simulink model "QCwithActDyn_seperate_channels"  (R2019b)
settings: Solver=FixedStepAuto  StartTime=0.0  StopTime=10  FixedStep=0.001  RelTol=1e-3
model workspace (MAT data in the model file):
  time_step = 0.01
libraries: simulink x1
settings Model: Creator=Abdulaziz Y. Alkayas  LastModifiedBy=aaa_b
settings SolverCC: SolverResetMethod=Robust
settings DebuggingCC: ArithmeticOperatorsInVariantConditions=warning
settings HardwareCC: TargetBitPerPointer=64  TargetBitPerSizeT=64  TargetBitPerPtrDiffT=64  TargetLongLongMode=on  TargetIntDivRoundTo=Zero  TargetEndianess=LittleEndian  TargetWordSize=64  TargetHWDeviceType=MATLAB Host  ProdEqTarget=off
settings SFSimCC: CustomCodeUndefinedFunction=UseInterfaceOnly
settings RTWCC: Description=Generic Real-Time Target

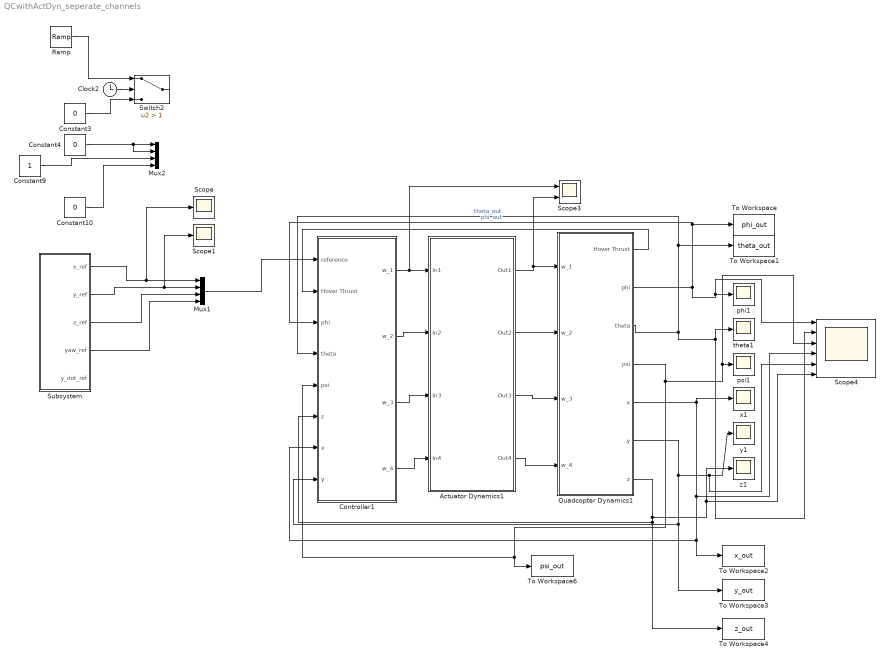
== system QCwithActDyn_seperate_channels ==
  Actuator Dynamics1 : Subsystem
  Clock2 : Clock
  Constant10 : Constant  Value=0
  Constant3 : Constant  Value=0
  Constant4 : Constant  Value=0
  Constant9 : Constant
  Controller1 : Subsystem
  Mux1 : Mux
  Mux2 : Mux
  Quadcopter Dynamics1 : Subsystem
  Ramp : simulink/Sources/Ramp  slope=1  start=2  InitialOutput=0
  Scope : Scope
  Scope1 : Scope
  Scope3 : Scope  NumInputPorts=2
  Scope4 : Scope  NumInputPorts=6
  Subsystem : Subsystem
  Switch2 : Switch  Criteria=u2 > Threshold  Threshold=1
  To Workspace : ToWorkspace  VariableName=phi_out  SaveFormat=Timeseries  SampleTime=-1
  To Workspace1 : ToWorkspace  VariableName=theta_out  SaveFormat=Timeseries  SampleTime=-1
  To Workspace2 : ToWorkspace  VariableName=x_out  SaveFormat=Timeseries  SampleTime=-1
  To Workspace3 : ToWorkspace  VariableName=y_out  SaveFormat=Timeseries  SampleTime=-1
  To Workspace4 : ToWorkspace  VariableName=z_out  SaveFormat=Timeseries  SampleTime=-1
  To Workspace6 : ToWorkspace  VariableName=psi_out  SaveFormat=Timeseries  SampleTime=-1
  phi1 : Scope
  psi1 : Scope
  theta1 : Scope
  x1 : Scope
  y1 : Scope
  z1 : Scope
  wires:
  Actuator Dynamics1/4(Out4) -> Quadcopter Dynamics1/4(w_4)
  Actuator Dynamics1/3(Out3) -> Quadcopter Dynamics1/3(w_3)
  Actuator Dynamics1/2(Out2) -> Quadcopter Dynamics1/2(w_2)
  Actuator Dynamics1/1(Out1) -> Scope3/2, Quadcopter Dynamics1/1(w_1)
  Controller1/4(w_4) -> Actuator Dynamics1/4(In4)
  Controller1/3(w_3) -> Actuator Dynamics1/3(In3)
  Controller1/2(w_2) -> Actuator Dynamics1/2(In2)
  Controller1/1(w_1) -> Actuator Dynamics1/1(In1), Scope3/1
  Quadcopter Dynamics1/3(theta) -> theta1/1, Scope4/2, To Workspace1/1, Controller1/4(theta)  "theta_out"
  Quadcopter Dynamics1/2(phi) -> Controller1/3(phi), To Workspace/1, phi1/1, Scope4/1  "phi_out"
  Quadcopter Dynamics1/4(psi) -> To Workspace6/1, Controller1/5(psi), psi1/1, Scope4/3
  Quadcopter Dynamics1/7(z) -> To Workspace4/1, Controller1/6(z), z1/1, Scope4/6
  Quadcopter Dynamics1/1(Hover Thrust) -> Controller1/2(Hover Thrust)
  Quadcopter Dynamics1/5(x) -> x1/1, Scope4/4, To Workspace2/1, Controller1/7(x)
  Quadcopter Dynamics1/6(y) -> To Workspace3/1, Controller1/8(y), y1/1, Scope4/5
  Ramp/1 -> Switch2/1
  Constant9/1 -> Mux2/3
  Constant10/1 -> Mux2/4
  Clock2/1 -> Switch2/2
  Constant3/1 -> Switch2/3
  Subsystem/3("z_ref ") -> Mux1/3
  Subsystem/4("yaw_ref ") -> Mux1/4
  Subsystem/1("x_ref ") -> Mux1/1, Scope/1
  Subsystem/2("y_ref ") -> Mux1/2, Scope1/1
  Constant4/1 -> Mux2/2, Mux2/1
  Mux1/1 -> Controller1/1(reference)

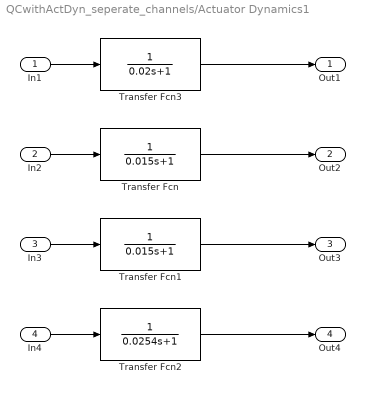
== system QCwithActDyn_seperate_channels/Actuator Dynamics1 ==
  In1 : Inport
  In2 : Inport  Port=2
  In3 : Inport  Port=3
  In4 : Inport  Port=4
  Transfer Fcn : TransferFcn  Denominator=[0.015 1]
  Transfer Fcn1 : TransferFcn  Denominator=[0.015 1]
  Transfer Fcn2 : TransferFcn  Denominator=[0.0254 1]
  Transfer Fcn3 : TransferFcn  Denominator=[0.02 1]
  Out1 : Outport
  Out2 : Outport  Port=2
  Out3 : Outport  Port=3
  Out4 : Outport  Port=4
  wires:
  In1/1 -> Transfer Fcn3/1
  In3/1 -> Transfer Fcn1/1
  Transfer Fcn3/1 -> Out1/1
  Transfer Fcn/1 -> Out2/1
  In2/1 -> Transfer Fcn/1
  Transfer Fcn1/1 -> Out3/1
  Transfer Fcn2/1 -> Out4/1
  In4/1 -> Transfer Fcn2/1

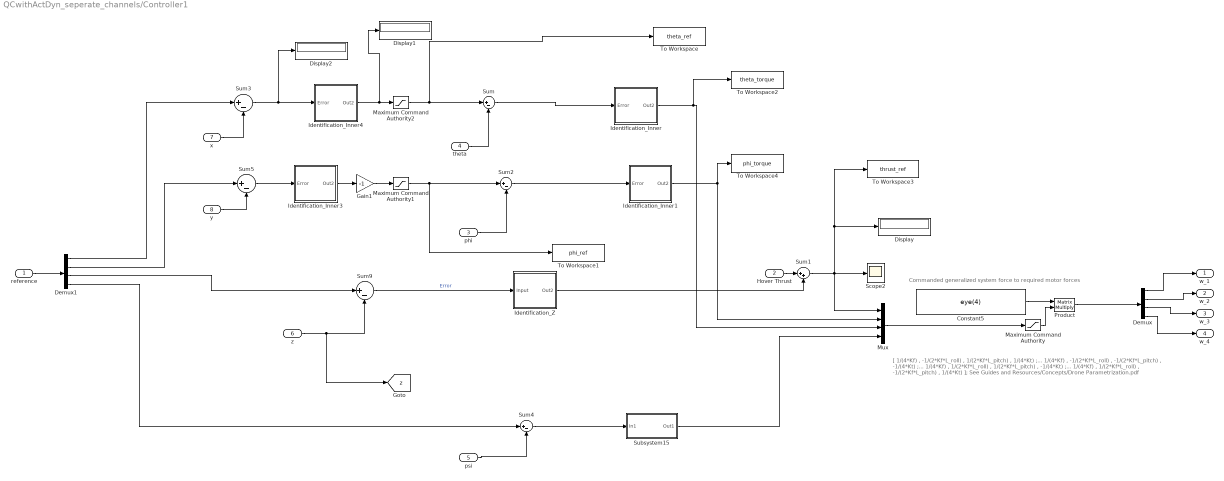
== system QCwithActDyn_seperate_channels/Controller1 ==
  note: [ 1/(4*Kf) , -1/(2*Kf*L_roll) , 1/(2*Kf*L_pitch) , 1/(4*Kt) ;...
      | 1/(4*Kf) , -1/(2*Kf*L_roll) , -1/(2*Kf*L_pitch) , -1/(4*Kt) ;...
      | 1/(4*Kf) , 1/(2*Kf*L_roll) , 1/(2*Kf*L_pitch) , -1/(4*Kt) ;...
      | 1/(4*Kf) , 1/(2*Kf*L_roll) , -1/(2*Kf*L_pitch) , 1/(4*Kt) ];
      |
      | See Guides and Resources/Concepts/Drone Parametrization.pdf
  note: Commanded generalized system force to required motor forces
  reference : Inport
  Hover Thrust : Inport  Port=2
  phi : Inport  Port=3
  theta : Inport  Port=4
  psi : Inport  Port=5
  z : Inport  Port=6
  x : Inport  Port=7
  y : Inport  Port=8
  Constant5 : Constant  Value=eye(4)
  Demux : Demux
  Demux1 : Demux
  Display : Display
  Display1 : Display
  Display2 : Display
  Gain1 : Gain  Gain=-1
  Identification_Inner : Subsystem
  Identification_Inner1 : Subsystem
  Identification_Inner3 : Subsystem
  Identification_Inner4 : Subsystem
  Identification_Z : Subsystem
  Maximum Command Authority : Saturate  UpperLimit=[Inf Inf Inf Inf]  LowerLimit=[-inf -Inf -Inf -Inf]
  Maximum Command Authority1 : Saturate  UpperLimit=pi/2  LowerLimit=-pi/2
  Maximum Command Authority2 : Saturate  UpperLimit=pi/2  LowerLimit=-pi/2
  Mux : Mux
  Product : Product  Multiplication=Matrix(*)
  Scope2 : Scope
  Subsystem15 : Subsystem
  Sum{,2..5,9} (6 alike) : Sum  Inputs=|+-
  Sum1 : Sum  Inputs=|++
  To Workspace : ToWorkspace  VariableName=theta_ref  SaveFormat=Timeseries  SampleTime=-1
  To Workspace1 : ToWorkspace  VariableName=phi_ref  SaveFormat=Timeseries  SampleTime=-1
  To Workspace2 : ToWorkspace  VariableName=theta_torque  SaveFormat=Timeseries  SampleTime=-1
  To Workspace3 : ToWorkspace  VariableName=thrust_ref  SaveFormat=Timeseries  SampleTime=-1
  To Workspace4 : ToWorkspace  VariableName=phi_torque  SaveFormat=Timeseries  SampleTime=-1
  w_1 : Outport
  w_2 : Outport  Port=2
  w_3 : Outport  Port=3
  w_4 : Outport  Port=4
  tag scope: z=global
  wires:
  Identification_Inner/1(Out2) -> To Workspace2/1, Mux/3
  Sum1/1 -> To Workspace3/1, Display/1, Scope2/1, Mux/1
  Subsystem15/1(Out1) -> Mux/4
  z/1 -> Sum9/2, [z]
  Identification_Inner1/1(Out2) -> Mux/2, To Workspace4/1
  Maximum Command Authority/1 -> Product/2
  Mux/1 -> Maximum Command Authority/1
  Constant5/1 -> Product/1
  Demux/2 -> w_2/1
  Demux/3 -> w_3/1
  Demux/4 -> w_4/1
  Sum3/1 -> Display2/1, Identification_Inner4/1(Error)
  Sum5/1 -> Identification_Inner3/1(Error)
  Hover Thrust/1 -> Sum1/1
  Demux/1 -> w_1/1
  Sum9/1 -> Identification_Z/1(Input)  "Error"
  Product/1 -> Demux/1
  Gain1/1 -> Maximum Command Authority1/1
  Maximum Command Authority1/1 -> Sum2/1, To Workspace1/1
  Maximum Command Authority2/1 -> To Workspace/1, Sum/1
  Identification_Z/1(Out2) -> Sum1/2
  reference/1 -> Demux1/1
  Demux1/3 -> Sum9/1
  Identification_Inner4/1(Out2) -> Maximum Command Authority2/1, Display1/1
  Identification_Inner3/1(Out2) -> Gain1/1
  x/1 -> Sum3/2
  y/1 -> Sum5/2
  Demux1/1 -> Sum3/1
  Demux1/2 -> Sum5/1
  Sum/1 -> Identification_Inner/1(Error)
  theta/1 -> Sum/2
  phi/1 -> Sum2/2
  Sum2/1 -> Identification_Inner1/1(Error)
  Sum4/1 -> Subsystem15/1(In1)
  psi/1 -> Sum4/2
  Demux1/4 -> Sum4/1

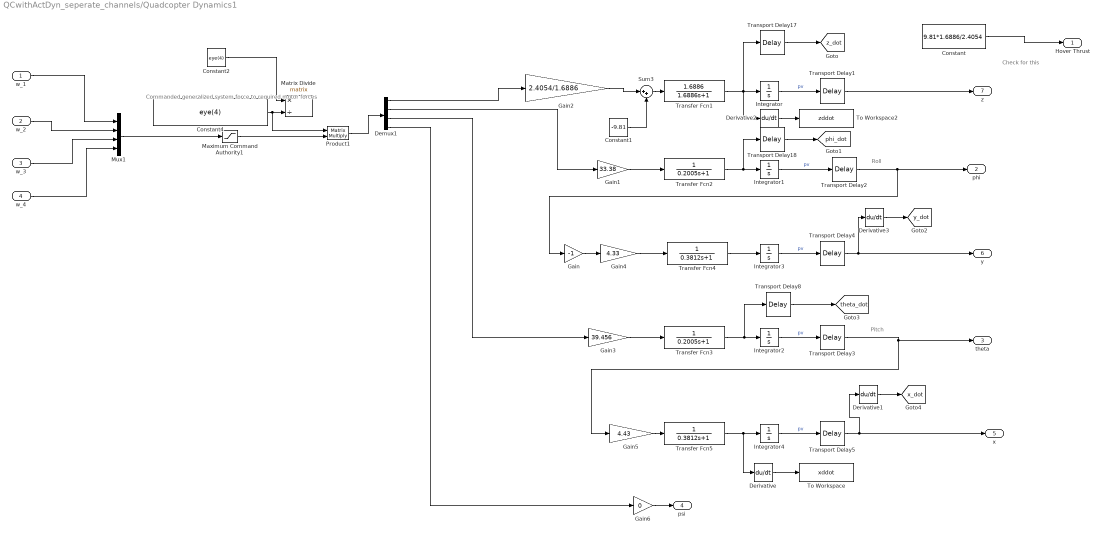
== system QCwithActDyn_seperate_channels/Quadcopter Dynamics1 ==
  note: Check for this
  note: Pitch
  note: Roll
  note: Commanded generalized system force to required motor forces
  w_1 : Inport
  w_2 : Inport  Port=2
  w_3 : Inport  Port=3
  w_4 : Inport  Port=4
  Constant : Constant  Value=9.81*1.6886/2.4054
  Constant1 : Constant  Value=-9.81
  Constant2 : Constant  Value=eye(4)
  Constant4 : Constant  Value=eye(4)
  Demux1 : Demux
  Derivative{,1..3} (4 alike) : Derivative
  Gain : Gain  Gain=-1
  Gain1 : Gain  Gain=33.38
  Gain2 : Gain  Gain=2.4054/1.6886
  Gain3 : Gain  Gain=39.456
  Gain4 : Gain  Gain=4.33
  Gain5 : Gain  Gain=4.43
  Gain6 : Gain  Gain=0
  Integrator{,1..4} (5 alike) : Integrator
  Matrix Divide : Product  Inputs=*/  Multiplication=Matrix(*)
  Maximum Command Authority1 : Saturate  UpperLimit=[Inf Inf Inf Inf]  LowerLimit=[-Inf -Inf -Inf -Inf]
  Mux1 : Mux
  Product1 : Product  Multiplication=Matrix(*)
  Sum3 : Sum  Inputs=|++
  To Workspace : ToWorkspace  VariableName=xddot  SaveFormat=Timeseries  SampleTime=-1
  To Workspace2 : ToWorkspace  VariableName=zddot  SaveFormat=Timeseries  SampleTime=-1
  Transfer Fcn1 : TransferFcn  Numerator=[1.6886]  Denominator=[1.6886 1]
  Transfer Fcn2 : TransferFcn  Denominator=[0.2005 1]
  Transfer Fcn3 : TransferFcn  Denominator=[0.2005 1]
  Transfer Fcn4 : TransferFcn  Denominator=[0.3812 1]
  Transfer Fcn5 : TransferFcn  Denominator=[0.3812 1]
  Transport Delay1 : TransportDelay  DelayTime=0.0237
  Transport Delay17 : TransportDelay  DelayTime=0.0237
  Transport Delay{2..3,8,18} (4 alike) : TransportDelay  DelayTime=0.025
  Transport Delay4 : TransportDelay  DelayTime=0.1
  Transport Delay5 : TransportDelay  DelayTime=0.1
  Hover Thrust : Outport
  phi : Outport  Port=2
  theta : Outport  Port=3
  psi : Outport  Port=4
  x : Outport  Port=5
  y : Outport  Port=6
  z : Outport  Port=7
  tag scope: phi_dot=global, theta_dot=global, x_dot=global, y_dot=global, z_dot=global
  wires:
  Transfer Fcn1/1 -> Derivative2/1, Transport Delay17/1, Integrator/1
  Integrator/1 -> Transport Delay1/1  "pv"
  Integrator1/1 -> Transport Delay2/1  "pv"
  Transfer Fcn2/1 -> Transport Delay18/1, Integrator1/1
  Gain1/1 -> Transfer Fcn2/1
  Transport Delay2/1 -> phi/1, Gain/1
  Gain3/1 -> Transfer Fcn3/1
  Transfer Fcn3/1 -> Transport Delay8/1, Integrator2/1
  Integrator2/1 -> Transport Delay3/1  "pv"
  Transport Delay3/1 -> theta/1, Gain5/1
  Demux1/2 -> Gain1/1
  Demux1/3 -> Gain3/1
  Integrator3/1 -> Transport Delay4/1  "pv"
  Gain5/1 -> Transfer Fcn5/1
  Transfer Fcn5/1 -> Derivative/1, Integrator4/1
  Sum3/1 -> Transfer Fcn1/1
  Integrator4/1 -> Transport Delay5/1  "pv"
  Demux1/4 -> Gain6/1
  w_2/1 -> Mux1/2
  w_3/1 -> Mux1/3
  w_4/1 -> Mux1/4
  Maximum Command Authority1/1 -> Product1/2
  Constant2/1 -> Matrix Divide/1
  Mux1/1 -> Maximum Command Authority1/1
  Constant4/1 -> Product1/1, Matrix Divide/2
  w_1/1 -> Mux1/1
  Demux1/1 -> Gain2/1
  Gain2/1 -> Sum3/1
  Gain/1 -> Gain4/1
  Transfer Fcn4/1 -> Integrator3/1
  Gain4/1 -> Transfer Fcn4/1
  Derivative/1 -> To Workspace/1
  Derivative2/1 -> To Workspace2/1
  Product1/1 -> Demux1/1
  Constant/1 -> Hover Thrust/1
  Transport Delay5/1 -> Derivative1/1, x/1
  Transport Delay8/1 -> [theta_dot]
  Transport Delay4/1 -> Derivative3/1, y/1
  Transport Delay1/1 -> z/1
  Transport Delay17/1 -> [z_dot]
  Transport Delay18/1 -> [phi_dot]
  Gain6/1 -> psi/1
  Derivative3/1 -> [y_dot]
  Constant1/1 -> Sum3/2
  Derivative1/1 -> [x_dot]

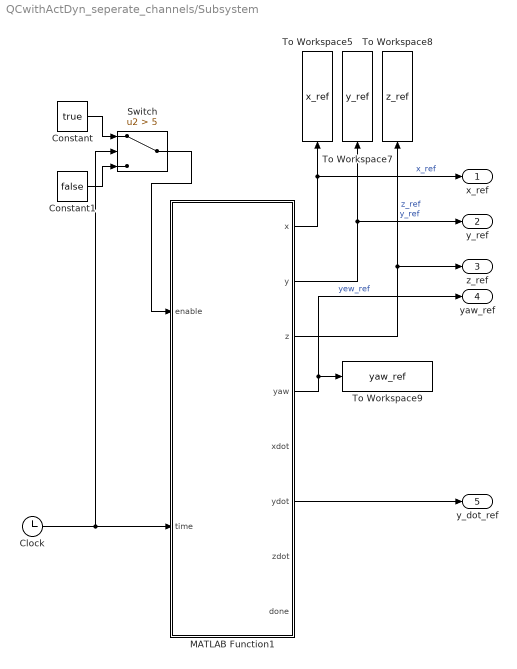
== system QCwithActDyn_seperate_channels/Subsystem ==
  Clock : Clock
  Constant : Constant  Value=true
  Constant1 : Constant  Value=false
  MATLAB Function1 : MATLAB Function  TreatAsAtomicUnit=on
  Switch : Switch  Criteria=u2 > Threshold  Threshold=5
  To Workspace5 : ToWorkspace  VariableName=x_ref  SaveFormat=Timeseries  SampleTime=-1
  To Workspace7 : ToWorkspace  VariableName=y_ref  SaveFormat=Timeseries  SampleTime=-1
  To Workspace8 : ToWorkspace  VariableName=z_ref  SaveFormat=Timeseries  SampleTime=-1
  To Workspace9 : ToWorkspace  VariableName=yaw_ref  SaveFormat=Timeseries  SampleTime=-1
  "x_ref " : Outport
  "y_ref " : Outport  Port=2
  "z_ref " : Outport  Port=3
  "yaw_ref " : Outport  Port=4
  "y_dot_ref " : Outport  Port=5
  wires:
  Switch/1 -> MATLAB Function1/1(enable)
  Clock/1 -> Switch/2, MATLAB Function1/2(time)
  MATLAB Function1/3(z) -> To Workspace8/1, "z_ref "/1  "z_ref"
  MATLAB Function1/1(x) -> "x_ref "/1, To Workspace5/1  "x_ref"
  MATLAB Function1/2(y) -> "y_ref "/1, To Workspace7/1  "y_ref"
  MATLAB Function1/4(yaw) -> "yaw_ref "/1, To Workspace9/1  "yew_ref"
  Constant/1 -> Switch/1
  Constant1/1 -> Switch/3
  MATLAB Function1/6(ydot) -> "y_dot_ref "/1

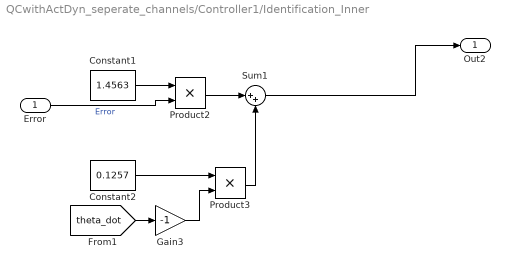
== system QCwithActDyn_seperate_channels/Controller1/Identification_Inner ==
  Error : Inport
  Constant1 : Constant  Value=1.4563
  Constant2 : Constant  Value=0.1257
  Gain3 : Gain  Gain=-1
  Product2 : Product
  Product3 : Product
  Sum1 : Sum  Inputs=|++
  Out2 : Outport
  wires:
  Error/1 -> Product2/2  "Error"
  [theta_dot] -> Gain3/1
  Product2/1 -> Sum1/1
  Constant2/1 -> Product3/1
  Gain3/1 -> Product3/2
  Constant1/1 -> Product2/1
  Sum1/1 -> Out2/1
  Product3/1 -> Sum1/2

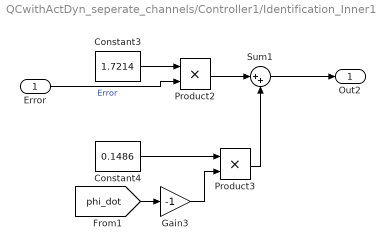
== system QCwithActDyn_seperate_channels/Controller1/Identification_Inner1 ==
  Error : Inport
  Constant3 : Constant  Value=1.7214
  Constant4 : Constant  Value=0.1486
  Gain3 : Gain  Gain=-1
  Product2 : Product
  Product3 : Product
  Sum1 : Sum  Inputs=|++
  Out2 : Outport
  wires:
  Sum1/1 -> Out2/1
  Product3/1 -> Sum1/2
  Constant4/1 -> Product3/1
  Constant3/1 -> Product2/1
  [phi_dot] -> Gain3/1
  Gain3/1 -> Product3/2
  Product2/1 -> Sum1/1
  Error/1 -> Product2/2  "Error"

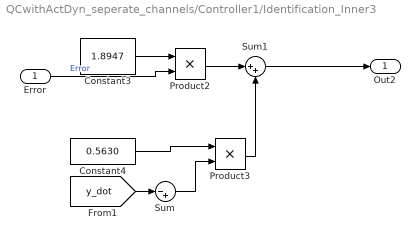
== system QCwithActDyn_seperate_channels/Controller1/Identification_Inner3 ==
  Error : Inport
  Constant3 : Constant  Value=1.8947
  Constant4 : Constant  Value=0.5630
  Product2 : Product
  Product3 : Product
  Sum : Sum  Inputs=|-+
  Sum1 : Sum  Inputs=|++
  Out2 : Outport
  wires:
  Error/1 -> Product2/2  "Error"
  [y_dot] -> Sum/1
  Product2/1 -> Sum1/1
  Constant4/1 -> Product3/1
  Sum/1 -> Product3/2
  Constant3/1 -> Product2/1
  Sum1/1 -> Out2/1
  Product3/1 -> Sum1/2

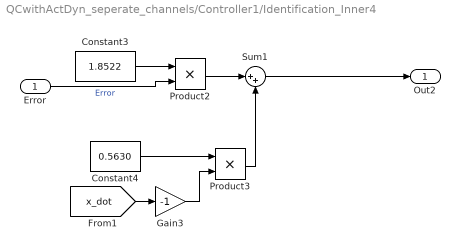
== system QCwithActDyn_seperate_channels/Controller1/Identification_Inner4 ==
  Error : Inport
  Constant3 : Constant  Value=1.8522
  Constant4 : Constant  Value=0.5630
  Gain3 : Gain  Gain=-1
  Product2 : Product
  Product3 : Product
  Sum1 : Sum  Inputs=|++
  Out2 : Outport
  wires:
  Error/1 -> Product2/2  "Error"
  [x_dot] -> Gain3/1
  Product2/1 -> Sum1/1
  Constant4/1 -> Product3/1
  Gain3/1 -> Product3/2
  Constant3/1 -> Product2/1
  Sum1/1 -> Out2/1
  Product3/1 -> Sum1/2

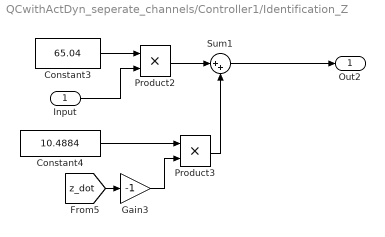
== system QCwithActDyn_seperate_channels/Controller1/Identification_Z ==
  Input : Inport
  Constant3 : Constant  Value=65.04
  Constant4 : Constant  Value=10.4884
  Gain3 : Gain  Gain=-1
  Product2 : Product
  Product3 : Product
  Sum1 : Sum  Inputs=|++
  Out2 : Outport
  wires:
  Constant4/1 -> Product3/1
  Sum1/1 -> Out2/1
  Gain3/1 -> Product3/2
  Product3/1 -> Sum1/2
  [z_dot] -> Gain3/1
  Product2/1 -> Sum1/1
  Constant3/1 -> Product2/1
  Input/1 -> Product2/2

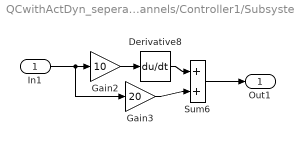
== system QCwithActDyn_seperate_channels/Controller1/Subsystem15 ==
  In1 : Inport
  Derivative8 : Derivative
  Gain2 : Gain  Gain=10
  Gain3 : Gain  Gain=20
  Sum6 : Sum  Inputs=|++
  Out1 : Outport
  wires:
  Gain2/1 -> Derivative8/1
  Gain3/1 -> Sum6/2
  Derivative8/1 -> Sum6/1
  Sum6/1 -> Out1/1
  In1/1 -> Gain3/1, Gain2/1

== matlab function QCwithActDyn_seperate_channels/Subsystem/MATLAB Function1 ==
  settings: updateMethod=DISCRETE
  data: enable input; x output; time input; y output; z output; yaw output; xdot output; ydot output; zdot output; done output
function [x, y, z, yaw, xdot, ydot, zdot, done]= fcn(enable, time)

persistent start_time
persistent poly_x
persistent poly_y
persistent poly_z
persistent n_order
persistent ts
persistent trajectory_segment
persistent state 
%states:
%   1: First trajectory
%   2: Second trajectory
%   3: Third trajectory


if isempty(start_time) || isempty(trajectory_segment) || ~enable || isempty(state)
    start_time = time;
    trajectory_segment = 1;
    state = 1;
end

% if isempty(poly_x) || isempty(poly_y) || isempty(poly_z) || isempty(ts)
%     g = coder.load('8shape-15_time_minsnap.mat');
%     poly_t = g.y;
%     n_order = g.poly_order;
%     ts = g.T;
% end
% 
% T = 5.5;
% x = 0; y = 0; z = 1; yaw=0; done=false;
% xdot = 0; ydot = 0; zdot = 0; 
% if enable
%     t = time - start_time;
%     if t > T
%         x = 0; y = 0; z = 1; yaw = 0; done = true;
%         xdot = 0; ydot = 0; zdot = 0; 
%         return;
%     end
%     t_now = 0;
%     for i=0:n_order-1
%         t_now = t_now + poly_t(i+1) * t^i;
%     end
%     t_now = 2*pi*t_now/T - pi/2;
%     x = 1*cos(t_now)*sin(t_now);
%     y = 1*cos(t_now);
%     
% end



% if isempty(poly_x) || isempty(poly_y) || isempty(poly_z) || isempty(ts)
%     g = coder.load('90_deg_roll24.mat');
%     poly_x = g.polys_x;
%     poly_y = g.polys_y;
%     poly_z = g.polys_z;
%     n_order = g.n_order(1);
%     ts = g.ts;
% end
% 
% x = -3; y = 0; z = 0.75; yaw=0; done=false;
% xdot = 0; ydot = 0; zdot = 0; 
% if enable
%     t = time - start_time;
%     if t > ts(end)
%         t=ts(end)
%     elseif t > ts(trajectory_segment + 1)
%         trajectory_segment = trajectory_segment + 1;
%     end
% 
% %     poly_x_i = poly_x(:, trajectory_segment);
% %     poly_y_i = poly_y(:, trajectory_segment);
% %     poly_z_i = poly_z(:, trajectory_segment);
%     poly_x_i = poly_x{trajectory_segment};
%     poly_y_i = poly_y{trajectory_segment};
%     poly_z_i = poly_z{trajectory_segment};
% 
%     x = 0; y = 0; z = 0.15;
%     for i=0:n_order
%         x = x + poly_x_i(i+1) * t^i;
%         y = y + poly_y_i(i+1) * t^i;
%         z = z + poly_z_i(i+1) * t^i;
%         if i>0
%             xdot = xdot + i * poly_x_i(i+1) * t^(i-1);
%             ydot = ydot + i * poly_y_i(i+1) * t^(i-1);
%             zdot = zdot + i * poly_z_i(i+1) * t^(i-1);
%         end
%     end
% end

% 
if isempty(poly_x) || isempty(poly_y) || isempty(poly_z) || isempty(n_order) || isempty(ts)
    g = coder.load('90_deg_roll24.mat');
    poly_x = g.polys_x;
    poly_y = g.polys_y;
    poly_z = g.polys_z;
    n_order = g.n_order(1);
    ts = g.ts;
end


x = -3; y = 0; z = 0.75; yaw=0; done=false;
xdot = 0; ydot = 0; zdot = 0; 
if enable
    t = time - start_time; 
    tt = t;
    if t > ts(end)
        tt = ts(end);
    elseif t > ts(trajectory_segment + 1)
        trajectory_segment = trajectory_segment + 1;
    end

%     poly_x_i = poly_x(:, trajectory_segment);
%     poly_y_i = poly_y(:, trajectory_segment);
%     poly_z_i = poly_z(:, trajectory_segment);
    poly_x_i = poly_x{trajectory_segment};
    poly_y_i = poly_y{trajectory_segment};
    poly_z_i = poly_z{trajectory_segment};

    offset = [0, 0, 0];
    if state == 1
        offset = [0, 0, 0.15];
    elseif state == 2
        offset = [0, 0, 0.15];
    elseif state == 3
        offset = [-0.25, 0.2, 0.25];
    end
    x = offset(1); y = offset(2); z = offset(3);
    for i=0:n_order
        x = x + poly_x_i(i+1) * tt^i;
        y = y + poly_y_i(i+1) * tt^i;
        z = z + poly_z_i(i+1) * tt^i;
        if i>0
            xdot = xdot + i * poly_x_i(i+1) * tt^(i-1);
            ydot = ydot + i * poly_y_i(i+1) * tt^(i-1);
            zdot = zdot + i * poly_z_i(i+1) * tt^(i-1);
        end
    end
    
    if t > ts(end)+0.5
        switch state
            case 1
                state = 2;
                start_time = time;
                g = coder.load('reset_traj_24_16.mat');
                poly_x = g.polys_x;
                poly_y = g.polys_y;
                poly_z = g.polys_z;
                n_order = g.n_order(1);
                ts = g.ts;
                trajectory_segment = 1;
            case 2
                if t > ts(end)+6
                    state = 3;
                    start_time = time;
                    g = coder.load('90_deg_roll16.mat');                
                    poly_x = g.polys_x;
                    poly_y = g.polys_y;
                    poly_z = g.polys_z;
                    n_order = g.n_order(1);
                    ts = g.ts;     
                    trajectory_segment = 1;       
                end
                
        end
    end
        
end
